simulink model "qAjustePID"  (Simulink 7.7)
settings: Solver=ode3  StartTime=0.0  StopTime=inf  FixedStep=0.02  RelTol=1e-3
libraries: simulink x7, aerolibfltsims x3, aerolibanimutils x1
settings Model: Creator=claus  LastModifiedBy=claus

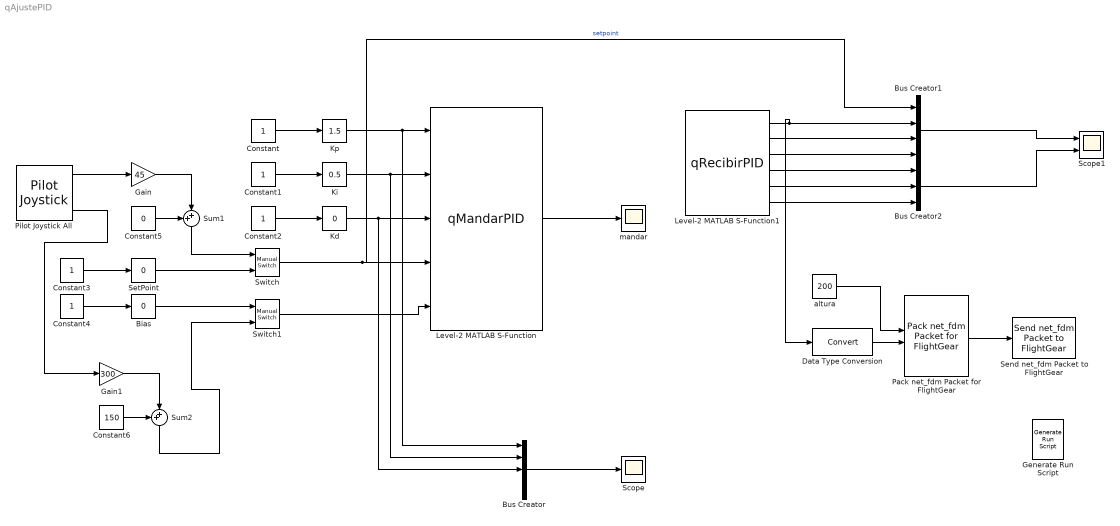
== system qAjustePID ==
  Bias : simulink/Math Operations/Slider Gain  SystemSampleTime=-1  low=0  gain=0  high=200
  Bus Creator : BusCreator  Inputs=5
  Bus Creator1 : BusCreator
  Bus Creator2 : BusCreator  Inputs=3
  Constant{,1..4} (5 alike) : Constant
  Constant5 : Constant  Value=0
  Constant6 : Constant  Value=150
  Data Type Conversion : DataTypeConversion
  Gain : Gain  Gain=45
  Gain1 : Gain  Gain=300
  Generate Run Script : aerolibfltsims/Generate Run Script  SystemSampleTime=-1  OutputFileName=runfg.bat  FlightGearBaseDirectory=C:\Program Files\FlightGear  GeometryModelName=QUADLSE  DestinationPort=5502  AirportId=LAX  RunwayId=1  InitialAltitude=200  InitialHeading=0  OffsetDistance=0  OffsetAzimuth=0  GenerateFile=off
  Kd : simulink/Math Operations/Slider Gain  SystemSampleTime=-1  low=0  gain=0  high=2
  Ki : simulink/Math Operations/Slider Gain  SystemSampleTime=-1  low=0  gain=0.5  high=5
  Kp : simulink/Math Operations/Slider Gain  SystemSampleTime=-1  low=0  gain=1.5  high=5
  Level-2 MATLAB S-Function : M-S-Function  FunctionName=qMandarPID  Parameters=host, puerto  mask(mandarPID){host='192.168.1.8', puerto=58887}
      mask prompts: host "Host (o 1 mostrar por consola)"
      mask help:
      | Manda los 4 parámetros de un controlador PID a través de un socket a un servidor corriendo en host:puerto.
      | Para mostrar la salida por la consola poner 1 en host.
      | El formato de salida se especifica en qFormatearPID_OUT.m
      mask Display:
      | port_label('input', 1, 'Kp');
      | port_label('input', 2, 'Ki');
      | port_label('input', 3, 'Kd');
      | port_label('input', 4, 'SetPoing');
      | port_label('input', 5, 'Bias');
      | port_label('output', 1, 'Mandar');
      | 
      | fprintf('qMandarPID');
  Level-2 MATLAB S-Function1 : M-S-Function  FunctionName=qRecibirPID  Parameters=host, port  mask{host='192.168.1.8', port=58888}
      mask prompts: port "Puerto"
      mask Display:
      | port_label('output', 1, 'valor 1')
      | port_label('output', 2, 'valor 2')
      | port_label('output', 3, 'valor 3')
      | port_label('output', 4, 'valor 4')
      | port_label('output', 5, 'valor 5')
      | port_label('output', 6, 'valor 6')
      | 
      | fprintf('qRecibirPID');
  Pack net_fdm Packet for FlightGear : aerolibfltsims/Pack net_fdm Packet for FlightGear  FlightGearVersion=v2.0  ShowPositionAttitudeInputs=on  ShowVelocityAccelerationInputs=off  ShowControlSurfacePositionInputs=off  ShowEngineFuelInputs=off  ShowLandingGearInputs=off  ShowEnvironmentInputs=off  SampleTime=-1
  Pilot Joystick All : aerolibanimutils/Pilot Joystick  JoystickID=Joystick1  OutputConfiguration=FourAxis  SampleTime=-1
  Scope : Scope
      settings: TimeRange=10  YMin=0  YMax=200
  Scope1 : Scope  NumInputPorts=2
      settings: TimeRange=10  YMin=-70~-225  YMax=60~75  SaveName=ScopeData2
  Send net_fdm Packet to FlightGear : aerolibfltsims/Send net_fdm Packet to FlightGear  DestinationIpAddress=127.0.0.1  DestinationPort=5502  LocalIpPort=-1  varLen=off  SampleTime=-1
  SetPoint : simulink/Math Operations/Slider Gain  SystemSampleTime=-1  low=0  gain=0  high=500
  Sum1 : Sum  Inputs=++|
  Sum2 : Sum  Inputs=++|
  Switch : simulink/Signal Routing/Manual Switch  SystemSampleTime=-1  sw=1  action=0  varsize=off
  Switch1 : simulink/Signal Routing/Manual Switch  SystemSampleTime=-1  sw=0  action=0  varsize=off
  altura : Constant  Value=200
  mandar : Scope
      settings: TimeRange=10  YMin=0  YMax=200
  wires:
  Constant/1 -> Kp/1
  Kp/1 -> Level-2 MATLAB S-Function/1, Bus Creator/1
  Constant1/1 -> Ki/1
  Ki/1 -> Level-2 MATLAB S-Function/2, Bus Creator/2
  Constant2/1 -> Kd/1
  Kd/1 -> Level-2 MATLAB S-Function/3, Bus Creator/3
  Bus Creator/1 -> Scope/1
  Constant4/1 -> Bias/1
  Constant3/1 -> SetPoint/1
  SetPoint/1 -> Switch/2
  Pilot Joystick All/1 -> Gain/1
  Gain/1 -> Sum1/2
  Sum1/1 -> Switch/1
  Constant5/1 -> Sum1/1
  Level-2 MATLAB S-Function/1 -> mandar/1
  Bus Creator1/1 -> Scope1/1
  Bus Creator2/1 -> Scope1/2
  Pack net_fdm Packet for FlightGear/1 -> Send net_fdm Packet to FlightGear/1
  Data Type Conversion/1 -> Pack net_fdm Packet for FlightGear/4
  altura/1 -> Pack net_fdm Packet for FlightGear/3
  Level-2 MATLAB S-Function1/4 -> Bus Creator2/1
  Bias/1 -> Switch1/1
  Switch1/1 -> Level-2 MATLAB S-Function/5
  Gain1/1 -> Sum2/2
  Sum2/1 -> Switch1/2
  Constant6/1 -> Sum2/1
  Pilot Joystick All/4 -> Gain1/1
  Switch/1 -> Bus Creator1/1, Level-2 MATLAB S-Function/4  "setpoint"
  Level-2 MATLAB S-Function1/1 -> Bus Creator1/2, Data Type Conversion/1
  Level-2 MATLAB S-Function1/3 -> Bus Creator1/4
  Level-2 MATLAB S-Function1/5 -> Bus Creator2/2
  Level-2 MATLAB S-Function1/6 -> Bus Creator2/3
  Level-2 MATLAB S-Function1/2 -> Bus Creator1/3
